simulink model "task3_MRAC3_finale"  (R2024b)
settings: Solver=VariableStepAuto  StartTime=0.0  StopTime=20  FixedStep=0.01  RelTol=1e-3
values from neighbouring files (symbols this model uses):
  F = [zeros(2,6);ones(1,6); row1; row2; direction * sigma]    [MAIN.m]    (also in MAIN_exam_2025.m)
  flag_PBMRAC = 0    [MAIN.m]
  lambda = diag(ones(6,1))*0.6    [MAIN.m]    (also in MAIN_exam_2025.m = diag(ones(6,1)))
  omegab_0 = [0 0 0]'    [MAIN.m]    (also in MAIN_exam_2025.m)
  p_0 = [17, 22.5, 0]'    [MAIN.m]    (also in MAIN_exam_2025.m = [0 0 0]')
  q_0 = eul2quat([0, theta_cmd, 0 ]*degToRad,'ZYX')'    [MAIN.m]    (also in MAIN_exam_2025.m = eul2quat([0, 0, 0 ]*degToRad,'XYZ')')
  stop_time = 80    [MAIN.m]    (also in MAIN_exam_2025.m = 20)
  traj =     [traiettoria_finale.mat]
  traj_case = 4    [MAIN.m]
  UAV = include_pack(UAV,pack,1)    [MAIN.m]
  vb_0 = zeros(3,1)    [MAIN.m]    (also in MAIN_exam_2025.m = [0 0 0]')
undefined symbols (not defined in the file or in its folder): adapt, ctrl, delay, min, par
libraries: matrix_library x2, aerolibutil x2, uavutilslib x1
settings Model: PacingRate=0.032000  Creator=ggera  LastModifiedBy=aurora
settings ConfigComp: CovBoundaryAbsTol=1.0e-5

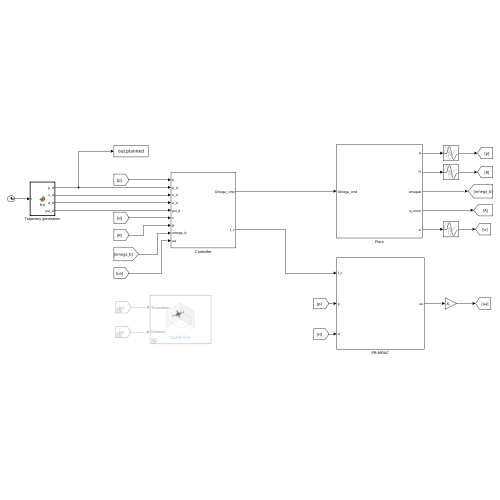
[thumbnail: Simulink's stored preview of the top-level diagram]
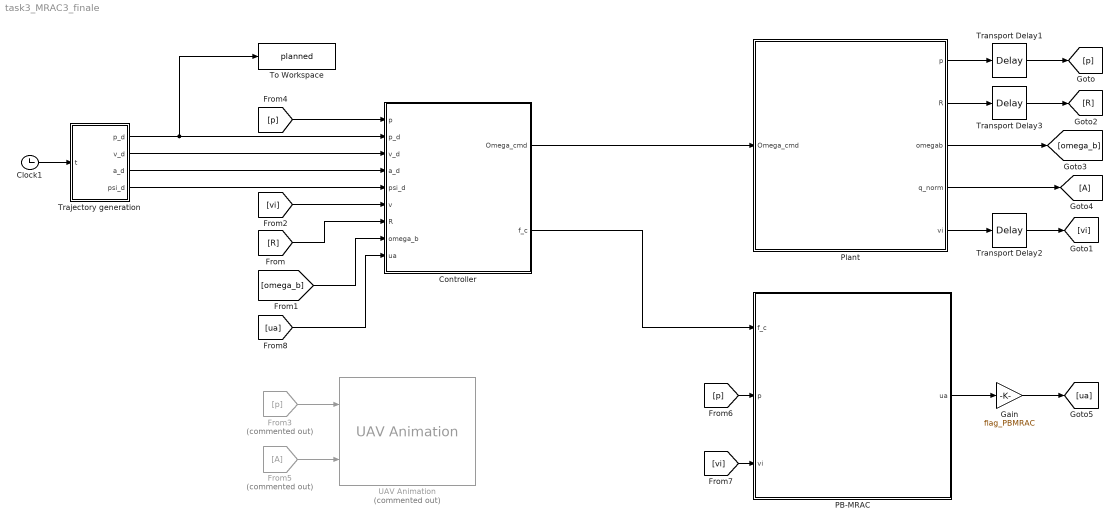
== system task3_MRAC3_finale ==
  Clock1 : Clock
  Controller : Subsystem
  From3 : From  Commented=on  GotoTag=p
  From5 : From  Commented=on
  Gain : Gain  Gain=flag_PBMRAC
  Goto4 : Goto
  PB-MRAC : Subsystem
  Plant : Subsystem
  To Workspace : ToWorkspace  VariableName=planned  SaveFormat=Timeseries  SampleTime=-1
  Trajectory generation : MATLAB Function  TreatAsAtomicUnit=on
  Transport Delay1 : TransportDelay  DelayTime=delay.position  InitialOutput=p_0
  Transport Delay2 : TransportDelay  DelayTime=delay.speed  InitialOutput=vb_0
  Transport Delay3 : TransportDelay  DelayTime=delay.attitude  InitialOutput=eye(3)
  UAV Animation : uavutilslib/UAV Animation  Commented=on  NumUAV=1  DynamicUAVConfig=off  UAVType=Multirotor  UAVSize=1  UAVColor=[1 0 0]  UAVTrajectoryAlpha=1  InertialZDirection=Up  RotationFormat=Quaternion  DrawMarkers=off  SampleTime=-1
  wires:
  Clock1/1 -> Trajectory generation/1(t)
  From3/1 -> UAV Animation/1
  From5/1 -> UAV Animation/2
  Trajectory generation/1(p_d) -> To Workspace/1, Controller/2(p_d)
  Trajectory generation/3(a_d) -> Controller/4(a_d)
  Trajectory generation/4(psi_d) -> Controller/5(psi_d)
  [vi] -> Controller/6(v)
  [R] -> Controller/7(R)
  [omega_b] -> Controller/8(omega_b)
  Plant/2(R) -> Transport Delay3/1
  Plant/3(omegab) -> [omega_b]
  Trajectory generation/2(v_d) -> Controller/3(v_d)
  [p] -> PB-MRAC/2(p)
  [vi] -> PB-MRAC/3(vi)
  [ua] -> Controller/9(ua)
  Controller/2(f_c) -> PB-MRAC/1(f_c)
  PB-MRAC/1(ua) -> Gain/1
  Controller/1(Omega_cmd) -> Plant/1(Omega_cmd)
  [p] -> Controller/1(p)
  Plant/1(p) -> Transport Delay1/1
  Plant/5(vi) -> Transport Delay2/1
  Transport Delay1/1 -> [p]
  Transport Delay2/1 -> [vi]
  Plant/4(q_norm) -> Goto4/1
  Transport Delay3/1 -> [R]
  Gain/1 -> [ua]

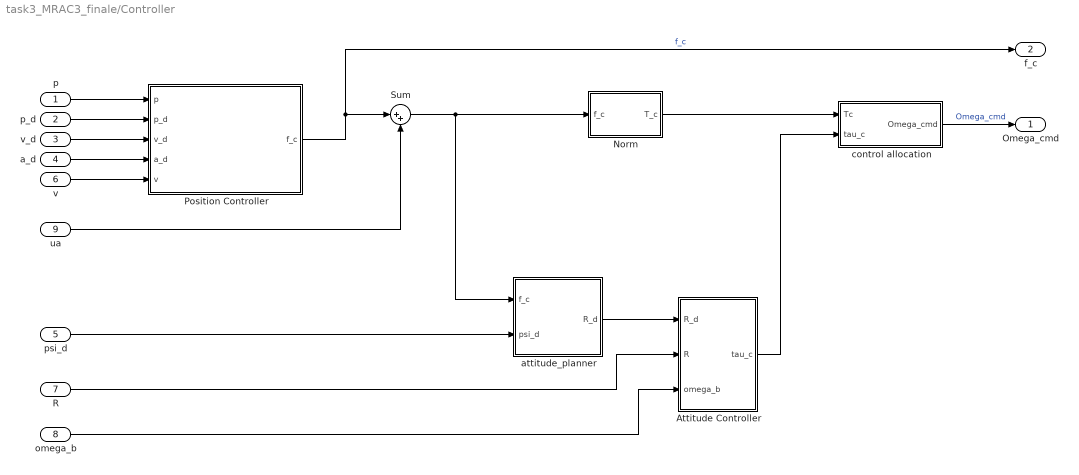
== system task3_MRAC3_finale/Controller ==
  p : Inport
  p_d : Inport  Port=2
  v_d : Inport  Port=3
  a_d : Inport  Port=4
  psi_d : Inport  Port=5
  v : Inport  Port=6
  R : Inport  Port=7
  omega_b : Inport  Port=8
  ua : Inport  Port=9
  Attitude Controller : Subsystem
  Norm : Subsystem
  Position Controller : Subsystem
  Sum : Sum  Inputs=|++
  attitude_planner : MATLAB Function  TreatAsAtomicUnit=on
  control allocation : Subsystem
  Omega_cmd : Outport
  f_c : Outport  Port=2
  wires:
  omega_b/1 -> Attitude Controller/3(omega_b)
  control allocation/1(Omega_cmd) -> Omega_cmd/1  "Omega_cmd"
  Attitude Controller/1(tau_c) -> control allocation/2(tau_c)
  v_d/1 -> Position Controller/3(v_d)
  a_d/1 -> Position Controller/4(a_d)
  attitude_planner/1(R_d) -> Attitude Controller/1(R_d)
  v/1 -> Position Controller/5(v)
  R/1 -> Attitude Controller/2(R)
  Norm/1(T_c) -> control allocation/1(Tc)
  p_d/1 -> Position Controller/2(p_d)
  p/1 -> Position Controller/1(p)
  psi_d/1 -> attitude_planner/2(psi_d)
  ua/1 -> Sum/2
  Position Controller/1(f_c) -> f_c/1, Sum/1  "f_c"
  Sum/1 -> Norm/1(f_c), attitude_planner/1(f_c)

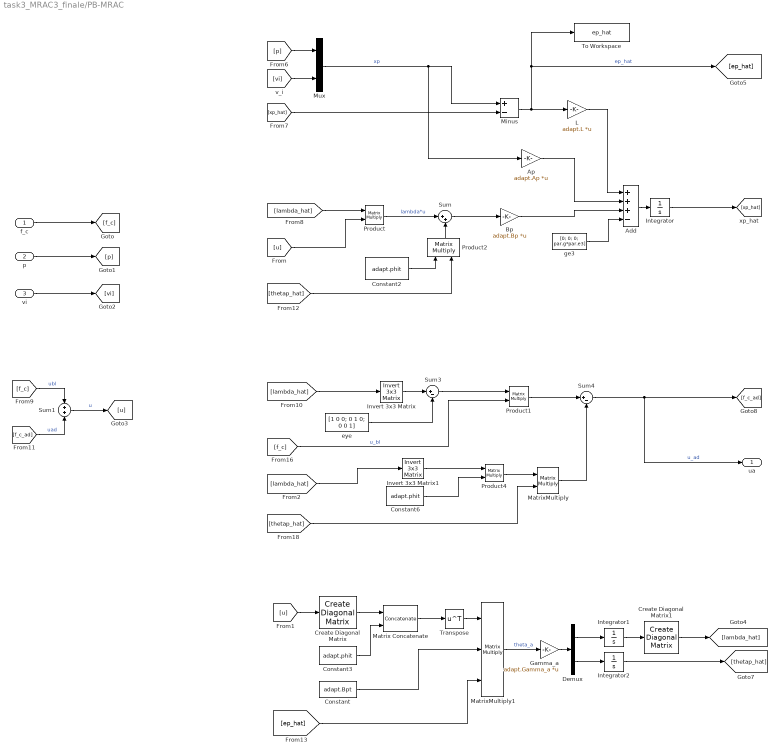
== system task3_MRAC3_finale/PB-MRAC ==
  f_c : Inport
  p : Inport  Port=2
  vi : Inport  Port=3
  Add : Sum  Inputs=+++-
  Ap : Gain  Gain=adapt.Ap  Multiplication=Matrix(K*u)
  Bp : Gain  Gain=adapt.Bp  Multiplication=Matrix(K*u)
  Constant : Constant  Value=adapt.Bpt
  Constant2 : Constant  Value=adapt.phit
  Constant3 : Constant  Value=adapt.phit
  Constant6 : Constant  Value=adapt.phit
  Create Diagonal Matrix : matrix_library/Create Diagonal Matrix
      settings: LibrarySourceBlock=|
      | simulink/Matrix
      | Operations/Create Diagonal
      | Matrix
  Create Diagonal Matrix1 : matrix_library/Create Diagonal Matrix
      settings: LibrarySourceBlock=|
      | simulink/Matrix
      | Operations/Create Diagonal
      | Matrix
  Demux : Demux  Outputs=2
  Gamma_a : Gain  Gain=adapt.Gamma_a  Multiplication=Matrix(K*u)
  Integrator : Integrator  InitialCondition=[p_0;vb_0]
  Integrator1 : Integrator  InitialCondition=[1;1;1]  LimitOutput=on  UpperSaturationLimit=1.3  LowerSaturationLimit=0.1
  Integrator2 : Integrator  InitialCondition=[0;0;0]  UpperSaturationLimit=3  LowerSaturationLimit=-3
  Invert 3x3 Matrix : aerolibutil/Invert  3x3 Matrix
  Invert 3x3 Matrix1 : aerolibutil/Invert  3x3 Matrix
  L : Gain  Gain=adapt.L  Multiplication=Matrix(K*u)
  Matrix Concatenate : Concatenate  Mode=Multidimensional array  ConcatenateDimension=2
  MatrixMultiply : Product  Multiplication=Matrix(*)
  MatrixMultiply1 : Product  Inputs=3  Multiplication=Matrix(*)
  Minus : Sum  Inputs=+-
  Mux : Mux  Inputs=2
  Product{,1..2,4} (4 alike) : Product  Inputs=**  Multiplication=Matrix(*)
  Sum : Sum  Inputs=|++
  Sum1 : Sum
  Sum3 : Sum  Inputs=|+-
  Sum4 : Sum  Inputs=|+-
  To Workspace : ToWorkspace  VariableName=ep_hat  SaveFormat=Timeseries  SampleTime=-1
  Transpose : Math  Operator=transpose
  eye : Constant  Value=[1 0 0; 0 1 0; 0 0 1]
  ge3 : Constant  Value=[0; 0; 0; par.g*par.e3]
  ua : Outport
  wires:
  Product1/1 -> Sum4/1
  Product2/1 -> Sum/2
  [lambda_hat] -> Invert 3x3 Matrix1/1
  Invert 3x3 Matrix1/1 -> Product4/1
  MatrixMultiply1/1 -> Gamma_a/1  "theta_a"
  Sum4/1 -> ua/1, [f_c_ad]  "u_ad"
  Sum/1 -> Bp/1
  [vi] -> Mux/2
  Invert 3x3 Matrix/1 -> Sum3/1
  [p] -> Mux/1
  Constant2/1 -> Product2/1
  [xp_hat] -> Minus/2
  Product/1 -> Sum/1  "lambda*u"
  [thetap_hat] -> Product2/2
  [lambda_hat] -> Product/1
  L/1 -> Add/1
  MatrixMultiply/1 -> Sum4/2
  Add/1 -> Integrator/1
  [thetap_hat] -> MatrixMultiply/2
  Mux/1 -> Ap/1, Minus/1  "xp"
  Sum3/1 -> Product1/1
  eye/1 -> Sum3/2
  [lambda_hat] -> Invert 3x3 Matrix/1
  Create Diagonal Matrix/1 -> Matrix Concatenate/1
  Minus/1 -> L/1, To Workspace/1, [ep_hat]  "ep_hat"
  f_c/1 -> [f_c]
  p/1 -> [p]
  vi/1 -> [vi]
  Ap/1 -> Add/2
  Bp/1 -> Add/3
  Demux/1 -> Integrator1/1
  Demux/2 -> Integrator2/1
  Transpose/1 -> MatrixMultiply1/1
  [ep_hat] -> MatrixMultiply1/3
  [u] -> Create Diagonal Matrix/1
  Gamma_a/1 -> Demux/1
  Integrator2/1 -> [thetap_hat]
  [f_c] -> Sum1/1  "ubl"
  Sum1/1 -> [u]  "u"
  [f_c_ad] -> Sum1/2  "uad"
  [f_c] -> Product1/2  "u_bl"
  Integrator1/1 -> Create Diagonal Matrix1/1
  Integrator/1 -> [xp_hat]
  Constant3/1 -> Matrix Concatenate/2
  Constant6/1 -> Product4/2
  Product4/1 -> MatrixMultiply/1
  Create Diagonal Matrix1/1 -> [lambda_hat]
  [u] -> Product/2
  Constant/1 -> MatrixMultiply1/2
  Matrix Concatenate/1 -> Transpose/1
  ge3/1 -> Add/4

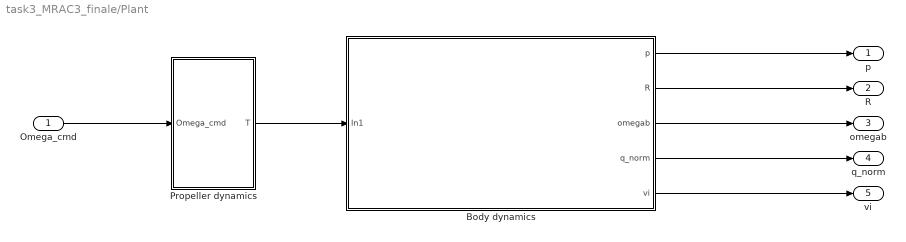
== system task3_MRAC3_finale/Plant ==
  Omega_cmd : Inport
  Body dynamics : Subsystem
  Propeller dynamics : Subsystem
  p : Outport
  R : Outport  Port=2
  omegab : Outport  Port=3
  q_norm : Outport  Port=4
  vi : Outport  Port=5
  wires:
  Propeller dynamics/1(T) -> Body dynamics/1(In1)
  Omega_cmd/1 -> Propeller dynamics/1(Omega_cmd)
  Body dynamics/2(R) -> R/1
  Body dynamics/1(p) -> p/1
  Body dynamics/3(omegab) -> omegab/1
  Body dynamics/5(vi) -> vi/1
  Body dynamics/4(q_norm) -> q_norm/1

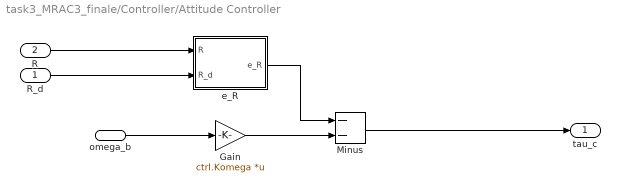
== system task3_MRAC3_finale/Controller/Attitude Controller ==
  R_d : Inport
  R : Inport  Port=2
  omega_b : Inport  Port=3
  Gain : Gain  Gain=ctrl.Komega  Multiplication=Matrix(K*u)
  Minus : Sum  Inputs=--
  "e_R " : MATLAB Function  TreatAsAtomicUnit=on
  tau_c : Outport
  wires:
  Minus/1 -> tau_c/1
  omega_b/1 -> Gain/1
  R/1 -> "e_R "/1(R)
  R_d/1 -> "e_R "/2(R_d)
  "e_R "/1(e_R) -> Minus/1
  Gain/1 -> Minus/2

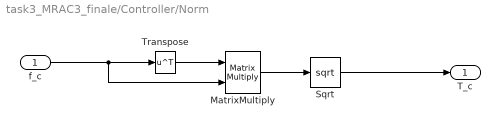
== system task3_MRAC3_finale/Controller/Norm ==
  f_c : Inport
  MatrixMultiply : Product  Multiplication=Matrix(*)
  Sqrt : Sqrt
  Transpose : Math  Operator=transpose
  T_c : Outport
  wires:
  f_c/1 -> MatrixMultiply/2, Transpose/1
  MatrixMultiply/1 -> Sqrt/1
  Sqrt/1 -> T_c/1
  Transpose/1 -> MatrixMultiply/1

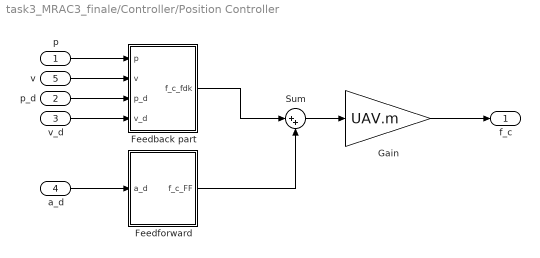
== system task3_MRAC3_finale/Controller/Position Controller ==
  p : Inport
  p_d : Inport  Port=2
  v_d : Inport  Port=3
  a_d : Inport  Port=4
  v : Inport  Port=5
  Feedback part : Subsystem
  Feedforward : Subsystem
  Gain : Gain  Gain=UAV.m
  Sum : Sum  Inputs=|++
  f_c : Outport
  wires:
  Gain/1 -> f_c/1
  p/1 -> Feedback part/1(p)
  Sum/1 -> Gain/1
  p_d/1 -> Feedback part/3(p_d)
  v/1 -> Feedback part/2(v)
  a_d/1 -> Feedforward/1(a_d)
  Feedforward/1(f_c_FF) -> Sum/2
  v_d/1 -> Feedback part/4(v_d)
  Feedback part/1(f_c_fdk) -> Sum/1

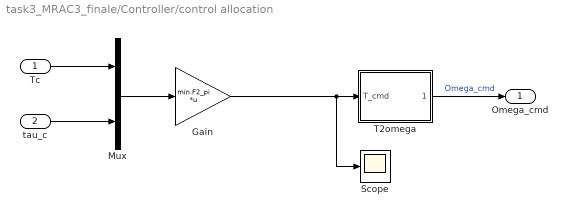
== system task3_MRAC3_finale/Controller/control allocation ==
  Tc : Inport
  tau_c : Inport  Port=2
  Gain : Gain  Gain=min.F2_pi  Multiplication=Matrix(K*u)
  Mux : Mux  Inputs=2
  Scope : Scope
  T2omega : MATLAB Function  TreatAsAtomicUnit=on
  Omega_cmd : Outport
  wires:
  T2omega/1(omega_cmd) -> Omega_cmd/1  "Omega_cmd"
  Mux/1 -> Gain/1
  tau_c/1 -> Mux/2
  Tc/1 -> Mux/1
  Gain/1 -> T2omega/1(T_cmd), Scope/1

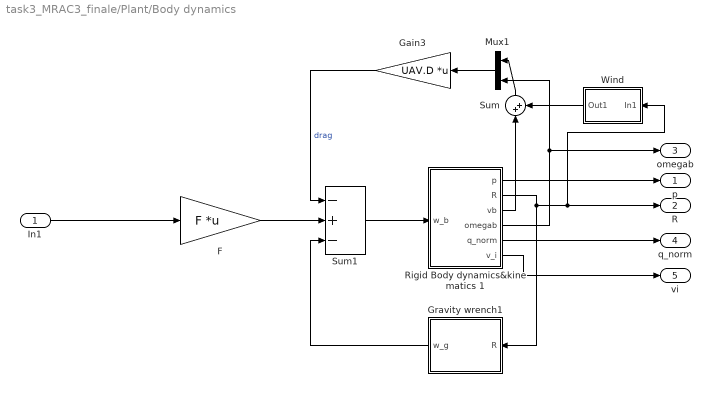
== system task3_MRAC3_finale/Plant/Body dynamics ==
  In1 : Inport
  F : Gain  Gain=F  Multiplication=Matrix(K*u)
  Gain3 : Gain  Gain=UAV.D  Multiplication=Matrix(K*u)
  Gravity wrench1 : MATLAB Function  TreatAsAtomicUnit=on
  Mux1 : Mux  Inputs=2
  Rigid Body dynamics&kinematics 1 : Subsystem
  Sum : Sum  Inputs=|++
  Sum1 : Sum  Inputs=-+-
  Wind : Subsystem
  p : Outport
  R : Outport  Port=2
  omegab : Outport  Port=3
  q_norm : Outport  Port=4
  vi : Outport  Port=5
  wires:
  Sum1/1 -> Rigid Body dynamics&kinematics 1/1(w_b)
  Mux1/1 -> Gain3/1
  Rigid Body dynamics&kinematics 1/4(omegab) -> Mux1/2, omegab/1
  Rigid Body dynamics&kinematics 1/2(R) -> Gravity wrench1/1(R), R/1, Wind/1(In1)
  Rigid Body dynamics&kinematics 1/1(p) -> p/1
  Rigid Body dynamics&kinematics 1/5(q_norm) -> q_norm/1
  Rigid Body dynamics&kinematics 1/6(v_i) -> vi/1
  In1/1 -> F/1
  Gain3/1 -> Sum1/1  "drag"
  F/1 -> Sum1/2
  Gravity wrench1/1(w_g) -> Sum1/3
  Rigid Body dynamics&kinematics 1/3(vb) -> Sum/1
  Sum/1 -> Mux1/1
  Wind/1(Out1) -> Sum/2

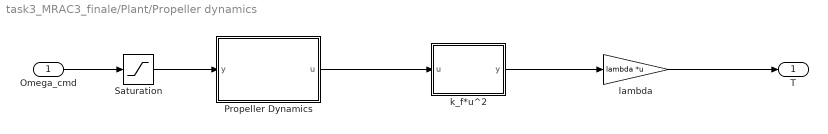
== system task3_MRAC3_finale/Plant/Propeller dynamics ==
  Omega_cmd : Inport
  Propeller Dynamics : Subsystem
  Saturation : Saturate  UpperLimit=UAV.Omega_max  LowerLimit=UAV.Omega_min
  k_f*u^2 : MATLAB Function  TreatAsAtomicUnit=on
  lambda : Gain  Gain=lambda  Multiplication=Matrix(K*u)
  T : Outport
  wires:
  Propeller Dynamics/1(u) -> k_f*u^2/1(u)
  k_f*u^2/1(y) -> lambda/1
  Omega_cmd/1 -> Saturation/1
  Saturation/1 -> Propeller Dynamics/1(y)
  lambda/1 -> T/1

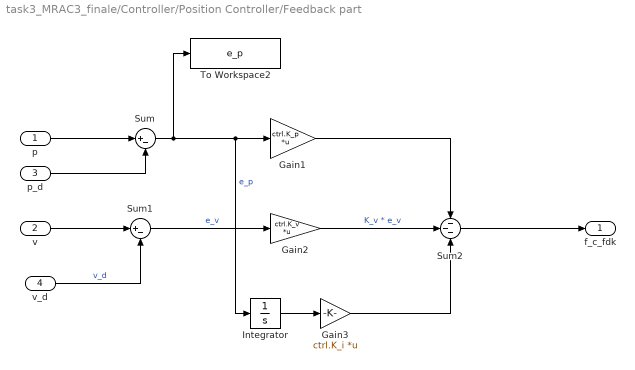
== system task3_MRAC3_finale/Controller/Position Controller/Feedback part ==
  p : Inport
  v : Inport  Port=2
  p_d : Inport  Port=3
  v_d : Inport  Port=4
  Gain1 : Gain  Gain=ctrl.K_p  Multiplication=Matrix(K*u)
  Gain2 : Gain  Gain=ctrl.K_v  Multiplication=Matrix(K*u)
  Gain3 : Gain  Gain=ctrl.K_i  Multiplication=Matrix(K*u)
  Integrator : Integrator
  Sum : Sum  Inputs=|+-
  Sum1 : Sum  Inputs=|+-
  Sum2 : Sum  Inputs=---
  To Workspace2 : ToWorkspace  VariableName=e_p  SaveFormat=Timeseries  SampleTime=-1
  f_c_fdk : Outport
  wires:
  p/1 -> Sum/1
  v_d/1 -> Sum1/2  "v_d"
  v/1 -> Sum1/1
  p_d/1 -> Sum/2
  Gain3/1 -> Sum2/3
  Integrator/1 -> Gain3/1
  Gain2/1 -> Sum2/2  "K_v * e_v"
  Sum1/1 -> Gain2/1  "e_v"
  Sum2/1 -> f_c_fdk/1
  Gain1/1 -> Sum2/1
  Sum/1 -> Gain1/1, Integrator/1, To Workspace2/1  "e_p"

== system task3_MRAC3_finale/Controller/Position Controller/Feedforward ==
  a_d : Inport
  Constant : Constant  Value=par.g*par.e3
  Sum3 : Sum
  f_c_FF : Outport
  wires:
  Sum3/1 -> f_c_FF/1
  a_d/1 -> Sum3/2
  Constant/1 -> Sum3/1

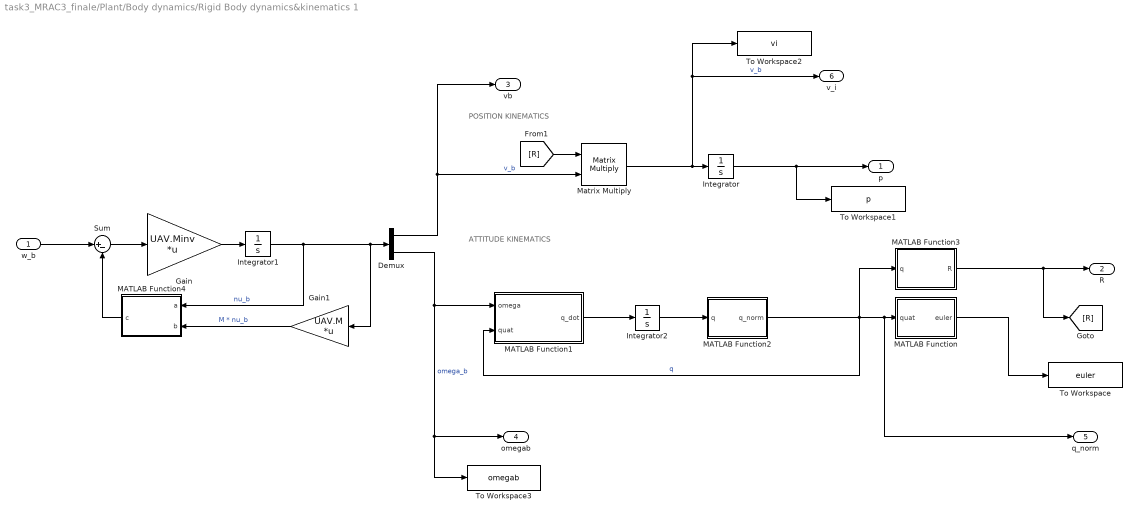
== system task3_MRAC3_finale/Plant/Body dynamics/Rigid Body dynamics&kinematics 1 ==
  note: POSITION KINEMATICS
  note: ATTITUDE KINEMATICS
  w_b : Inport
  Demux : Demux  Outputs=2
  Gain : Gain  Gain=UAV.Minv  Multiplication=Matrix(K*u)
  Gain1 : Gain  Gain=UAV.M  Multiplication=Matrix(K*u)
  Integrator : Integrator  InitialCondition=p_0
  Integrator1 : Integrator  InitialCondition=[vb_0;omegab_0]
  Integrator2 : Integrator  InitialCondition=q_0
  MATLAB Function : MATLAB Function  TreatAsAtomicUnit=on
  MATLAB Function1 : MATLAB Function  TreatAsAtomicUnit=on
  MATLAB Function2 : MATLAB Function  TreatAsAtomicUnit=on
  MATLAB Function3 : MATLAB Function  TreatAsAtomicUnit=on
  MATLAB Function4 : MATLAB Function  TreatAsAtomicUnit=on
  Matrix Multiply : Product  Multiplication=Matrix(*)
  Sum : Sum  Inputs=|+-
  To Workspace : ToWorkspace  VariableName=euler  SaveFormat=Timeseries  SampleTime=-1
  To Workspace1 : ToWorkspace  VariableName=p  SaveFormat=Timeseries  SampleTime=-1
  To Workspace2 : ToWorkspace  VariableName=vi  SaveFormat=Timeseries  SampleTime=-1
  To Workspace3 : ToWorkspace  VariableName=omegab  SaveFormat=Timeseries  SampleTime=-1
  p : Outport
  R : Outport  Port=2
  vb : Outport  Port=3
  omegab : Outport  Port=4
  q_norm : Outport  Port=5
  v_i : Outport  Port=6
  wires:
  w_b/1 -> Sum/1
  MATLAB Function4/1(c) -> Sum/2
  Sum/1 -> Gain/1
  Gain1/1 -> MATLAB Function4/2(b)  "M * nu_b"
  Demux/2 -> MATLAB Function1/1(omega), To Workspace3/1, omegab/1  "omega_b"
  Gain/1 -> Integrator1/1
  [R] -> Matrix Multiply/1
  MATLAB Function/1(euler) -> To Workspace/1
  Integrator2/1 -> MATLAB Function2/1(q)
  Integrator1/1 -> MATLAB Function4/1(a), Gain1/1, Demux/1  "nu_b"
  Demux/1 -> Matrix Multiply/2, vb/1  "v_b"
  MATLAB Function3/1(R) -> [R], R/1
  MATLAB Function2/1(q_norm) -> MATLAB Function3/1(q), q_norm/1, MATLAB Function/1(quat), MATLAB Function1/2(quat)  "q"
  MATLAB Function1/1(q_dot) -> Integrator2/1
  Matrix Multiply/1 -> v_i/1, To Workspace2/1, Integrator/1  "v_b"
  Integrator/1 -> To Workspace1/1, p/1

== system task3_MRAC3_finale/Plant/Body dynamics/Wind ==
  In1 : Inport
  MatrixMultiply : Product  Multiplication=Matrix(*)
  Transpose : Math  Operator=transpose
  Wind : Step  Time=0  After=adapt.wind  SampleTime=0  VectorParams1D=off
  Out1 : Outport
  wires:
  Wind/1 -> MatrixMultiply/2
  MatrixMultiply/1 -> Out1/1
  Transpose/1 -> MatrixMultiply/1
  In1/1 -> Transpose/1

== system task3_MRAC3_finale/Plant/Propeller dynamics/Propeller Dynamics ==
  y : Inport
  Gain : Gain  Gain=-UAV.k_m
  Integrator : Integrator  InitialCondition=zeros(6,1)
  Sum1 : Sum  Inputs=|-+
  u : Outport
  wires:
  Gain/1 -> Integrator/1
  y/1 -> Sum1/1
  Integrator/1 -> u/1, Sum1/2  "Omega"
  Sum1/1 -> Gain/1

== matlab function task3_MRAC3_finale/Plant/Body dynamics/Gravity wrench1 ==
  data: R input; w_g output; UAV parameter; par parameter
function w_g = fcn(R,UAV,par)

e_3 = par.e3;
g = par.g;

w_g = g*[UAV.m*R'*e_3; UAV.S*R'*e_3];

== matlab function task3_MRAC3_finale/Controller/attitude_planner ==
  data: f_c input; R_d output; psi_d input
function R_d = fcn(f_c,psi_d)
% fc expected: coloumn vector

hd = [cos(psi_d), sin(psi_d), 0]';
kp = f_c./norm(f_c);
jp = cross(kp,hd)/norm(cross(kp, hd));
ip = cross(jp, kp);
R_d = [ip, jp, kp];

== matlab function task3_MRAC3_finale/Trajectory generation ==
  data: t input; p_d output; v_d output; a_d output; psi_d output; traj parameter; stop_time parameter; traj_case parameter
function [p_d,v_d,a_d, psi_d] = fcn(t,traj,stop_time,traj_case)

psi_d = deg2rad(0);
p_d = zeros(3,1);
v_d = zeros(3,1); 
a_d = zeros(3,1); 
tttt = traj;
switch traj_case
    case 1
        
        %circular trajectory
        Omega_d= 1; % rad/s
        R_d=1; % m
        
        p_d = R_d*[cos(Omega_d*t) sin(Omega_d*t) 1]';
        v_d = R_d*Omega_d*[-sin(Omega_d*t) cos(Omega_d*t) 0]';
        a_d = -R_d*Omega_d^2*[cos(Omega_d*t) sin(Omega_d*t) 0]';
        
    case 2 

        % setpoint tracking
        p_d = [1;1 ; 1];
        v_d = zeros(3,1); 
        a_d = zeros(3,1); 
    
    case 3
    
        % Sinusoidal trajectory
        A = 1.0;        
        omega = 1;   
        v_y = 0.5;      
        z_d = 1;      
        x = A * sin(omega * t);     
        y = v_y * t;               
        z = z_d;
        p_d = [x; y; z];
        x_dot = A * omega * cos(omega * t);
        y_dot = v_y;
        z_dot = 0;
        v_d = [x_dot; y_dot; z_dot];
        x_ddot = -A * omega^2 * sin(omega * t);
        y_ddot = 0;
        z_ddot = 0;

       a_d = [x_ddot; y_ddot; z_ddot];
    
    case 4
        
        % delivery scenario
        p_d = [17; 22.5 ; 3/10*t];
        v_d = [0 0 0]'; 
        a_d = [0 0 0]'; 
        
        time = [traj.t 60]; 
        
        if t > 10 && t < 70
             px = interp1(time,[traj.pd(1,:) traj.pd(1,end)],t-10); 
             py = interp1(time,[traj.pd(2,:) traj.pd(2,end)],t-10);
             pz = interp1(time,[traj.pd(3,:) traj.pd(3,end)],t-10);
        
             vx = interp1(time,[traj.vd(1,:) traj.vd(1,end)],t-10); 
             vy = interp1(time,[traj.vd(2,:) traj.vd(2,end)],t-10);
             vz = interp1(time,[traj.vd(3,:) traj.vd(3,end)],t-10);
        
             ax = interp1(time,[traj.ad(1,:) traj.ad(1,end)],t-10); 
             ay = interp1(time,[traj.ad(2,:) traj.ad(2,end)],t-10);
             az = interp1(time,[traj.ad(3,:) traj.ad(3,end)],t-10);
        
             p_d = [px;py;pz];
             v_d = [vx;vy;vz];
             a_d = [ax;ay;az];
        elseif t > 70
            p_d = [-12; -12.5 ; 3/10*(stop_time-t)];
            v_d = [0 0 0]'; 
            a_d = zeros(3,1); 
        
        end
end

== matlab function task3_MRAC3_finale/Plant/Propeller dynamics/k_f*u^2 ==
  data: u input; y output; k_f parameter
function y = T(u, k_f)
    y = u;
    a = length(u);
    for i = 1:a
        y(i) = k_f * u(i)^2;
    end
end

== matlab function task3_MRAC3_finale/Controller/Attitude Controller/e_R  ==
  data: R input; e_R output; R_d input; par parameter
function e_R = fcn(R,R_d,par) 
k_R1 = par.k_R1; 
k_R2 = par.k_R2; 
k_R3 = par.k_R3; 

e_1 = [1 0 0]';
e_2 = [0 1 0]';
e_3 = [0 0 1]';

R_e = R_d' * R;
e_R = k_R1 * cross(R_e' * e_1,e_1) + k_R2 * cross(R_e' * e_2,e_2) + k_R3 * cross(R_e' * e_3,e_3);

== matlab function task3_MRAC3_finale/Controller/control allocation/T2omega ==
  data: T_cmd input; omega_cmd output; k_f parameter
function omega_cmd = fcn(T_cmd,k_f)

omega_cmd = sqrt(T_cmd/k_f);

== matlab function task3_MRAC3_finale/Plant/Body dynamics/Rigid Body dynamics&kinematics 1/MATLAB Function ==
  data: quat input; euler output
function euler = quatToEuler( quat )
%	Converts a quaternion vector to ZYX Euler angles (RPY)

euler = quat2eul(quat','ZYX');

end

== matlab function task3_MRAC3_finale/Plant/Body dynamics/Rigid Body dynamics&kinematics 1/MATLAB Function1 ==
  data: omega input; quat input; q_dot output
 function q_dot = quat_kin(omega, quat)
%#codegen

eta = quat(1);
eps = quat(2:4);

W=[-eps';
   skew(eps) + eta*eye(3)];

q_dot = 0.5*W*omega;

end

function S=skew(s)
S=[0  -s(3)  s(2);
    s(3)   0 -s(1);
    -s(2)  s(1)  0];
end

== matlab function task3_MRAC3_finale/Plant/Body dynamics/Rigid Body dynamics&kinematics 1/MATLAB Function2 ==
  data: q input; q_norm output
function q_norm = quat_norm( q )

norm = sqrt( q(1)^2 + q(2)^2 + q(3)^2 + q(4)^2 );

q_norm = 1/norm * q;

== matlab function task3_MRAC3_finale/Plant/Body dynamics/Rigid Body dynamics&kinematics 1/MATLAB Function3 ==
  data: q input; R output
function R = fcn(q)

R = quat2rotm(q');

end

== matlab function task3_MRAC3_finale/Plant/Body dynamics/Rigid Body dynamics&kinematics 1/MATLAB Function4 ==
  data: a input; c output; b input
function c = cross_six(a,b)

a_v = a(1:3);
a_omega = a(4:6);

cross_six = [crossmat(a_omega), zeros(3,3);
             crossmat(a_v), crossmat(a_omega)] ;

c = cross_six*b;

end

function S=crossmat(s)
S=[0  -s(3)  s(2);
    s(3)   0 -s(1);
    -s(2)  s(1)  0];
end
